simulink model "msfun_test"  (R2013a)
settings: Solver=FixedStepDiscrete  StartTime=0.0  StopTime=10.0  FixedStep=0.1  RelTol=1e-3
settings Model: Creator=luca  LastModifiedBy=luca

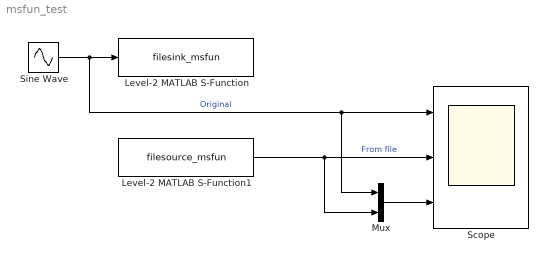
== system msfun_test ==
  Level-2 MATLAB S-Function : M-S-Function  FunctionName=filesink_msfun  Parameters='testfile'
  Level-2 MATLAB S-Function1 : M-S-Function  FunctionName=filesource_msfun  Parameters='testfile' 0
  Mux : Mux  Inputs=2
  Scope : Scope  NumInputPorts=3
      settings: TimeRange=10  YMin=-5~-5~-5  YMax=5~5~5
  Sine Wave : Sin  SampleTime=0
  wires:
  Sine Wave/1 -> Level-2 MATLAB S-Function/1, Mux/1, Scope/1  "Original"
  Level-2 MATLAB S-Function1/1 -> Mux/2, Scope/2  "From file"
  Mux/1 -> Scope/3
